simulink model "dcBusPITuning"  (R2025b)
settings: Solver=ode4  StartTime=0.0  StopTime=1.0  FixedStep=0.001  RelTol=1e-3
libraries: simulink x1, slpidlib x1
settings Model: Creator=Santhosh  LastModifiedBy=Santhosh

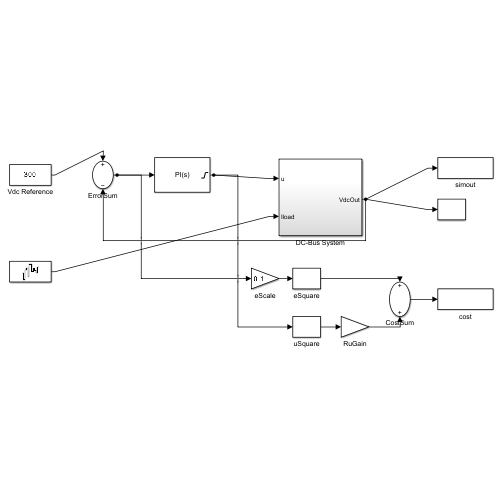
[thumbnail: Simulink's stored preview of the top-level diagram]
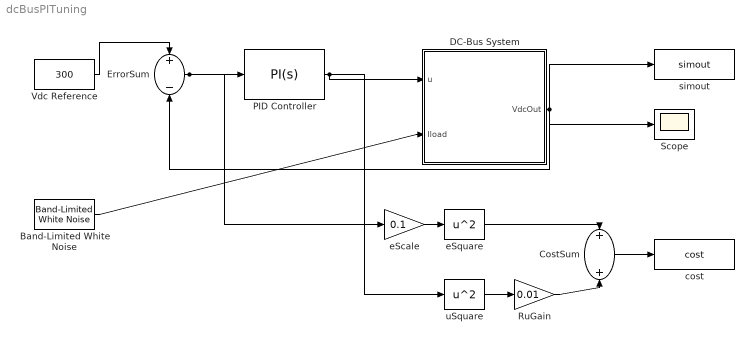
== system dcBusPITuning ==
  Band-Limited White Noise : simulink/Sources/Band-Limited White Noise  Cov=5  Ts=0.001  seed=23341
  CostSum : Sum
  DC-Bus System : Subsystem
  ErrorSum : Sum  Inputs=+-
  PID Controller : slpidlib/PID Controller  Controller=PI  Form=Parallel  TimeDomain=Continuous-time  UseExternalTs=off  SampleTime=-1  IntegratorMethod=Forward Euler  FilterMethod=Forward Euler  ControllerParametersSource=internal  P=0.075567  I=0.64811  UseKiTs=off  D=0  UseExternalDerivativeSource=off  N=100  UseFilter=on  TunerSelectOption=Transfer Function Based (PID Tuner App)  InitialConditionSource=internal  InitialConditionForIntegrator=0  InitialConditionForFilter=0  DifferentiatorICPrevScaledInput=0  ExternalReset=none  TrackingMode=off  Kt=1  LimitOutput=on  SatLimitsSource=internal  UpperSaturationLimit=10.0503  LowerSaturationLimit=-9.3339  LinearizeAsGain=on  AntiWindupMode=clamping  Kb=1  LimitIntegrator=off  UpperIntegratorSaturationLimit=inf  LowerIntegratorSaturationLimit=-inf  POutMin=[]  POutMax=[]  IOutMin=[]  IOutMax=[]  DOutMin=[]  DOutMax=[]  NOutMin=[]  NOutMax=[]  SumOutMin=[]  SumOutMax=[]  SaturationOutMin=[]  SaturationOutMax=[]  PParamMin=[]  PParamMax=[]  IParamMin=[]  IParamMax=[]  DParamMin=[]  DParamMax=[]  NParamMin=[]  NParamMax=[]  KbParamMin=[]  KbParamMax=[]  KtParamMin=[]  KtParamMax=[]  KbOutMin=[]  KbOutMax=[]  KtOutMin=[]  KtOutMax=[]  IntegratorOutMin=[]  IntegratorOutMax=[]  FilterOutMin=[]  FilterOutMax=[]  SumI1OutMin=[]  SumI1OutMax=[]  SumI2OutMin=[]  SumI2OutMax=[]  SumI3OutMin=[]  SumI3OutMax=[]  SumI4OutMin=[]  SumI4OutMax=[]  SumDOutMin=[]  SumDOutMax=[]  DifferentiatorOutMin=[]  DifferentiatorOutMax=[]  FilterDiffOutCoefMin=[]  FilterDiffOutCoefMax=[]  ReciprocalOutMin=[]  ReciprocalOutMax=[]  SumDenOutMin=[]  SumDenOutMax=[]  SumNumOutMin=[]  SumNumOutMax=[]  DivideOutMin=[]  DivideOutMax=[]  UdiffTsProdOutMin=[]  UdiffTsProdOutMax=[]  NTsProdOutMin=[]  NTsProdOutMax=[]  UintegralTsProdOutMin=[]  UintegralTsProdOutMax=[]  UngainTsProdOutMin=[]  UngainTsProdOutMax=[]  ClampingZeroOutDataTypeStr=Inherit: Inherit via back propagation  ClampingZeroOutMin=[]  ClampingZeroOutMax=[]  FilterDenConstantOutDataTypeStr=Inherit: Inherit via back propagation  FilterDenConstantOutMin=[]  FilterDenConstantOutMax=[]  PCopyOutDataTypeStr=Inherit: Inherit via back propagation  PCopyOutMin=[]  PCopyOutMax=[]  NCopyOutDataTypeStr=Inherit: Inherit via back propagation  NCopyOutMin=[]  NCopyOutMax=[]  IntegratorContinuousStateAttributes=''  IntegratorStateMustResolveToSignalObject=off  IntegratorRTWStateStorageClass=Auto  FilterContinuousStateAttributes=''  FilterStateMustResolveToSignalObject=off  FilterRTWStateStorageClass=Auto  ParallelPVariant=InternalParameters  IdealPVariant=Disabled  IVariant=InternalParameters  DVariant=Disabled  IntegratorVariant=Continuous  SatVariant=Enabled  AWVariant=ContClampingParallel  PCopyVariant=Disabled  TRVariant=Disabled  FdbkBlocksVariant=Forward  IdealPFdbkVariant=Disabled  SatFdbkVariant=Disabled  DerivativeFilterVariant=Disabled  NVariant=Disabled  NCopyVariant=Disabled_SignalSpec  FilterICVariant=Disabled  IntegratorICVariant=InternalICs  ExternalResetVariant=Disabled  TRSumVariant=Passthrough  SumFdbkVariant=Disabled  SumVariant=Sum_PI  TsampFilterVariant=InternalTs  TsampNgainVariant=Passthrough  TsampIntegralVariant=Disabled_SignalSpec  ExternalSaturationOutDataTypeStr=Inherit: Same as second input  DerivativeSourceVariant=Disabled  PreIntVariant=InternalPreInt
  RuGain : Gain  Gain=0.01
  Scope : Scope
  Vdc Reference : Constant  Value=300
  cost : ToWorkspace  VariableName=cost  SaveFormat=Timeseries  SampleTime=-1
  eScale : Gain  Gain=0.1
  eSquare : Math  Operator=square
  simout : ToWorkspace  VariableName=simout  SaveFormat=Timeseries  SampleTime=-1
  uSquare : Math  Operator=square
  wires:
  Vdc Reference/1 -> ErrorSum/1
  ErrorSum/1 -> PID Controller/1, eScale/1
  PID Controller/1 -> DC-Bus System/1(u), uSquare/1
  Band-Limited White Noise/1 -> DC-Bus System/2(Iload)
  DC-Bus System/1(VdcOut) -> simout/1, Scope/1, ErrorSum/2
  eScale/1 -> eSquare/1
  uSquare/1 -> RuGain/1
  eSquare/1 -> CostSum/1
  RuGain/1 -> CostSum/2
  CostSum/1 -> cost/1

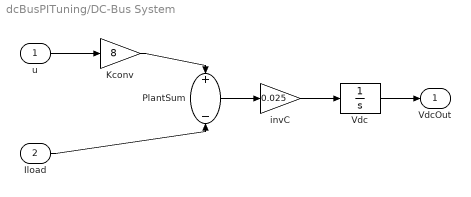
== system dcBusPITuning/DC-Bus System ==
  u : Inport
  Iload : Inport  Port=2
  Kconv : Gain  Gain=8
  PlantSum : Sum  Inputs=+-
  Vdc : Integrator  InitialCondition=297.9049
  invC : Gain  Gain=0.025
  VdcOut : Outport
  wires:
  u/1 -> Kconv/1
  Kconv/1 -> PlantSum/1
  Iload/1 -> PlantSum/2
  PlantSum/1 -> invC/1
  invC/1 -> Vdc/1
  Vdc/1 -> VdcOut/1
